simulink model "wheel_speed_control_19a"  (R2019a)
settings: Solver=VariableStepAuto  StartTime=0.0  StopTime=10.0  RelTol=1e-3  EnableMultiTasking=on
undefined symbols (not defined in the file or in its folder): d, i_1, i_2, K_T, T
settings Model: Creator=TFRICKE  LastModifiedBy=YUMU
settings DataIOCC: LimitDataPoints=on  ReturnWorkspaceOutputs=off
settings OptimizationCC: LifeSpan=inf
settings DebuggingCC: AllowSymbolicDim=off  SFUnexpectedBacktrackingDiag=warning  SFNoUnconditionalDefaultTransitionDiag=warning  SFExecutionAtInitializationDiag=none  ArithmeticOperatorsInVariantConditions=warning
settings ModelReferenceCC: PropagateSignalLabelsOutOfModel=off
settings SFSimCC: SimUseLocalCustomCode=off
settings RTWCC: RTWUseLocalCustomCode=off
settings CodeAppCC: StateflowObjectComments=on
settings GRTTargetCC: TargetLangStandard=C89/C90 (ANSI)
settings ConfigComp: CovMetricSettings=dw  CovHtmlReporting=on  CovSaveCumulativeToWorkspaceVar=on  CovSaveSingleToWorkspaceVar=on  CovExternalEMLEnable=off

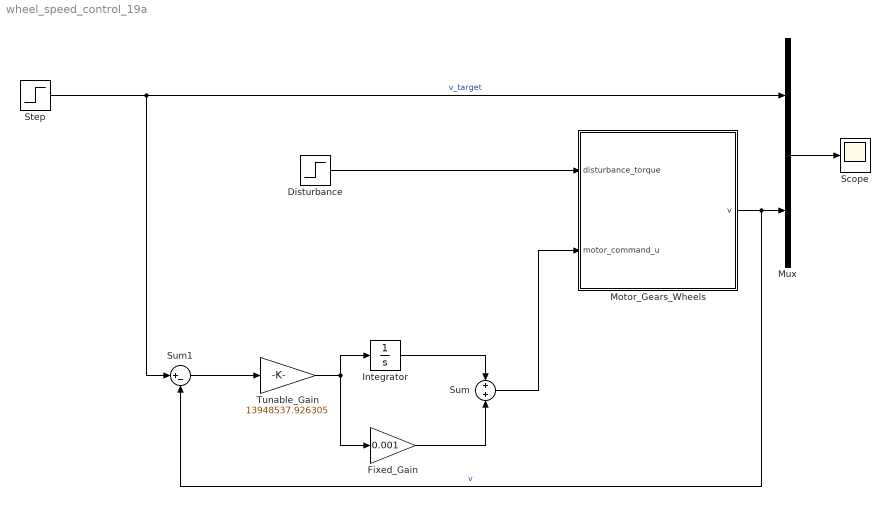
== system wheel_speed_control_19a ==
  Disturbance : Step  Time=5  After=-300  SampleTime=0
  Fixed_Gain : Gain  Gain=0.001
  Integrator : Integrator
  Motor_Gears_Wheels : Subsystem
  Mux : Mux  Inputs=2
  Scope : Scope
  Step : Step  SampleTime=0
  Sum : Sum
  Sum1 : Sum  Inputs=|+-
  Tunable_Gain : Gain  Gain=13948537.926305
  wires:
  Motor_Gears_Wheels/1(v) -> Sum1/2, Mux/2  "v"
  Step/1 -> Sum1/1, Mux/1  "v_target"
  Disturbance/1 -> Motor_Gears_Wheels/1(disturbance_torque)
  Mux/1 -> Scope/1
  Tunable_Gain/1 -> Integrator/1, Fixed_Gain/1
  Integrator/1 -> Sum/1
  Fixed_Gain/1 -> Sum/2
  Sum1/1 -> Tunable_Gain/1
  Sum/1 -> Motor_Gears_Wheels/2(motor_command_u)

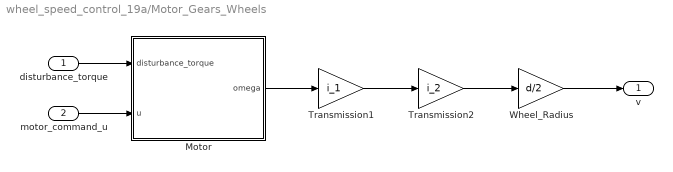
== system wheel_speed_control_19a/Motor_Gears_Wheels ==
  disturbance_torque : Inport
  motor_command_u : Inport  Port=2
  Motor : Subsystem
  Transmission1 : Gain  Gain=i_1
  Transmission2 : Gain  Gain=i_2
  Wheel_Radius : Gain  Gain=d/2
  v : Outport  VectorParamsAs1DForOutWhenUnconnected=off
  wires:
  Transmission2/1 -> Wheel_Radius/1
  Transmission1/1 -> Transmission2/1
  Motor/1(omega) -> Transmission1/1
  motor_command_u/1 -> Motor/2(u)
  Wheel_Radius/1 -> v/1
  disturbance_torque/1 -> Motor/1(disturbance_torque)

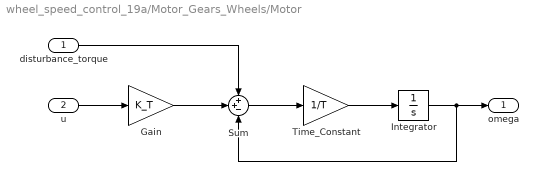
== system wheel_speed_control_19a/Motor_Gears_Wheels/Motor ==
  disturbance_torque : Inport
  u : Inport  Port=2
  Gain : Gain  Gain=K_T
  Integrator : Integrator
  Sum : Sum  Inputs=++-
  Time_Constant : Gain  Gain=1/T
  omega : Outport  VectorParamsAs1DForOutWhenUnconnected=off
  wires:
  Gain/1 -> Sum/2
  Integrator/1 -> Sum/3, omega/1
  Sum/1 -> Time_Constant/1
  Time_Constant/1 -> Integrator/1
  u/1 -> Gain/1
  disturbance_torque/1 -> Sum/1
